simulink model "UAV_Autotune_Model_4Axis"  (R2024b)
settings: Solver=ode23t  StartTime=0.0  StopTime=55  MaxStep=0.01  RelTol=1e-3
values from neighbouring files (symbols this model uses):
  P = merge_struct_recursive(P,A.overrides)    [apply_aircraft_definition.m]    (also in uav_actuator_sfunc.m = block.DialogPrm(1).Data; uav_aero_sfunc.m = block.DialogPrm(1).Data; uav_autopilot_sfunc.m = block.DialogPrm(1).Data; uav_command_sfunc.m = block.DialogPrm(1).Data)
libraries: aerolibatmos2 x1, aerolibobsolete x1, shared6dof x1
settings Model: Creator=dell  LastModifiedBy=dell

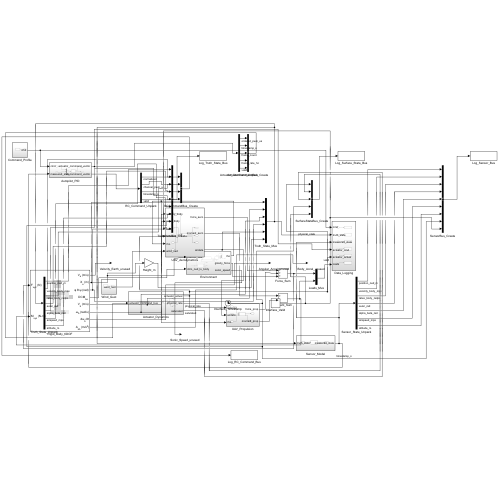
[thumbnail: Simulink's stored preview of the top-level diagram]
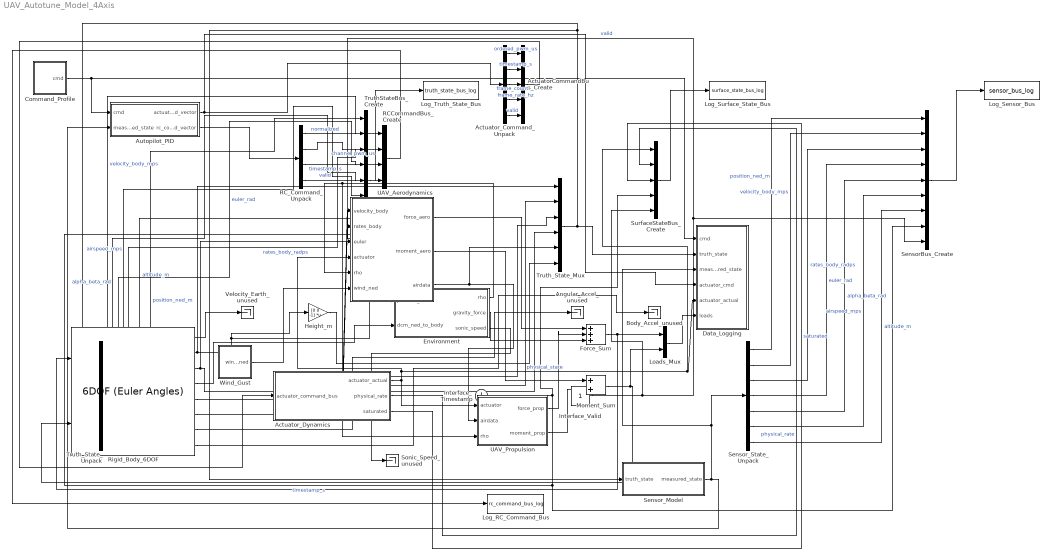
== system UAV_Autotune_Model_4Axis ==
  ActuatorCommandBus_Create : BusCreator  Inputs=5  OutDataTypeStr=Bus: ActuatorCommandBus
  Actuator_Command_Unpack : Demux  Outputs=[5 1 1 1 1]
  Actuator_Dynamics : Subsystem
  Angular_Accel_unused : Terminator
  Autopilot_PID : Subsystem
  Body_Accel_unused : Terminator
  Command_Profile : Subsystem
  Data_Logging : Subsystem
  Environment : Subsystem
  Force_Sum : Sum  Inputs=+++
  Height_m : Gain  Gain=[0 0 -1]  Multiplication=Matrix(K*u)
  Interface_Timestamp : Clock
  Interface_Valid : Constant
  Loads_Mux : Mux  Inputs=2
  Log_RC_Command_Bus : ToWorkspace  VariableName=rc_command_bus_log  SaveFormat=Timeseries  SampleTime=-1
  Log_Sensor_Bus : ToWorkspace  VariableName=sensor_bus_log  SaveFormat=Timeseries  SampleTime=-1
  Log_Surface_State_Bus : ToWorkspace  VariableName=surface_state_bus_log  SaveFormat=Timeseries  SampleTime=-1
  Log_Truth_State_Bus : ToWorkspace  VariableName=truth_state_bus_log  SaveFormat=Timeseries  SampleTime=-1
  Moment_Sum : Sum
  RCCommandBus_Create : BusCreator  Inputs=4  OutDataTypeStr=Bus: RCCommandBus
  RC_Command_Unpack : Demux  Outputs=[4 8 1 1]
  Rigid_Body_6DOF : shared6dof/6DOF (Euler Angles)  units=Metric (MKS)  mtype=Fixed  rep=Euler Angles  xme_0=P.init.position_ned  Vm_0=P.init.velocity_body  eul_0=P.init.euler  pm_0=P.init.body_rates  mass_0=P.mass  mass_e=0.5  mass_f=2.0  inertia=P.inertia  inertia_e=eye(3)  inertia_f=2*eye(3)  k_quat=1.0  vre_flag=on  abi_flag=off  aMode=aMode  xme_statename=''  Vm_statename=''  eul_statename=''  quat_statename=''  pm_statename=''  mass_statename=''
  SensorBus_Create : BusCreator  Inputs=9  OutDataTypeStr=Bus: SensorBus
  Sensor_Model : Subsystem
  Sensor_State_Unpack : Demux  Outputs=[3 3 3 3 2 1 1]
  Sonic_Speed_unused : Terminator
  SurfaceStateBus_Create : BusCreator  Inputs=5  OutDataTypeStr=Bus: SurfaceStateBus
  TruthStateBus_Create : BusCreator  Inputs=9  OutDataTypeStr=Bus: TruthStateBus
  Truth_State_Mux : Mux  Inputs=6
  Truth_State_Unpack : Demux  Outputs=[3 3 3 3 2 1 1]
  UAV_Aerodynamics : Subsystem
  UAV_Propulsion : Subsystem
  Velocity_Earth_unused : Terminator
  Wind_Gust : Subsystem
  wires:
  Loads_Mux/1 -> Data_Logging/6(loads)
  Command_Profile/1(cmd) -> Autopilot_PID/1(cmd), Data_Logging/1(cmd)
  Rigid_Body_6DOF/8 -> Body_Accel_unused/1
  Rigid_Body_6DOF/7 -> Angular_Accel_unused/1
  Rigid_Body_6DOF/1 -> Velocity_Earth_unused/1
  Rigid_Body_6DOF/3 -> Truth_State_Mux/4, UAV_Aerodynamics/3(euler)
  Rigid_Body_6DOF/6 -> Truth_State_Mux/3, UAV_Aerodynamics/2(rates_body)
  Rigid_Body_6DOF/5 -> Truth_State_Mux/2, UAV_Aerodynamics/1(velocity_body)
  Rigid_Body_6DOF/4 -> Environment/2(dcm_ned_to_body)
  Rigid_Body_6DOF/2 -> Height_m/1, Environment/1(position_ned), Truth_State_Mux/1
  Environment/1(rho) -> UAV_Aerodynamics/5(rho), UAV_Propulsion/3(rho)
  UAV_Aerodynamics/3(airdata) -> Truth_State_Mux/5, UAV_Propulsion/2(airdata)
  UAV_Aerodynamics/1(force_aero) -> Force_Sum/1
  UAV_Propulsion/1(force_prop) -> Force_Sum/2
  Environment/2(gravity_force) -> Force_Sum/3
  UAV_Aerodynamics/2(moment_aero) -> Moment_Sum/1
  UAV_Propulsion/2(moment_prop) -> Moment_Sum/2
  Height_m/1 -> Truth_State_Mux/6
  Force_Sum/1 -> Rigid_Body_6DOF/1, Loads_Mux/1
  Moment_Sum/1 -> Rigid_Body_6DOF/2, Loads_Mux/2
  Environment/3(sonic_speed) -> Sonic_Speed_unused/1
  RC_Command_Unpack/4 -> RCCommandBus_Create/4  "valid"
  RC_Command_Unpack/3 -> RCCommandBus_Create/3  "timestamp_s"
  Autopilot_PID/2(rc_command_vector) -> RC_Command_Unpack/1
  RC_Command_Unpack/1 -> RCCommandBus_Create/1  "normalized"
  RC_Command_Unpack/2 -> RCCommandBus_Create/2  "channel_pwm_us"
  SensorBus_Create/1 -> Log_Sensor_Bus/1
  Sensor_State_Unpack/7 -> SensorBus_Create/7  "altitude_m"
  Sensor_State_Unpack/6 -> SensorBus_Create/6  "airspeed_mps"
  Sensor_State_Unpack/5 -> SensorBus_Create/5  "alpha_beta_rad"
  Sensor_State_Unpack/4 -> SensorBus_Create/4  "euler_rad"
  Sensor_State_Unpack/3 -> SensorBus_Create/3  "rates_body_radps"
  Sensor_State_Unpack/2 -> SensorBus_Create/2  "velocity_body_mps"
  Sensor_State_Unpack/1 -> SensorBus_Create/1  "position_ned_m"
  TruthStateBus_Create/1 -> Log_Truth_State_Bus/1
  Truth_State_Unpack/7 -> TruthStateBus_Create/7  "altitude_m"
  Truth_State_Unpack/6 -> TruthStateBus_Create/6  "airspeed_mps"
  Truth_State_Unpack/5 -> TruthStateBus_Create/5  "alpha_beta_rad"
  Truth_State_Unpack/4 -> TruthStateBus_Create/4  "euler_rad"
  Truth_State_Unpack/3 -> TruthStateBus_Create/3  "rates_body_radps"
  Truth_State_Unpack/2 -> TruthStateBus_Create/2  "velocity_body_mps"
  Truth_State_Unpack/1 -> TruthStateBus_Create/1  "position_ned_m"
  SurfaceStateBus_Create/1 -> Log_Surface_State_Bus/1
  Interface_Valid/1 -> SensorBus_Create/9, TruthStateBus_Create/9, SurfaceStateBus_Create/5  "valid"
  Interface_Timestamp/1 -> SensorBus_Create/8, TruthStateBus_Create/8, SurfaceStateBus_Create/4  "timestamp_s"
  Actuator_Dynamics/3(saturated) -> SurfaceStateBus_Create/3  "saturated"
  Actuator_Dynamics/2(physical_rate) -> SurfaceStateBus_Create/2  "physical_rate"
  RCCommandBus_Create/1 -> Log_RC_Command_Bus/1
  ActuatorCommandBus_Create/1 -> Actuator_Dynamics/1(actuator_command_bus)
  Actuator_Command_Unpack/2 -> ActuatorCommandBus_Create/2  "timestamp_s"
  Actuator_Command_Unpack/1 -> ActuatorCommandBus_Create/1  "ordered_pwm_us"
  Actuator_Dynamics/1(actuator_actual) -> SurfaceStateBus_Create/1, Data_Logging/5(actuator_actual), UAV_Aerodynamics/4(actuator), UAV_Propulsion/1(actuator)  "physical_state"
  Autopilot_PID/1(actuator_command_vector) -> Actuator_Command_Unpack/1, Data_Logging/4(actuator_cmd)
  Actuator_Command_Unpack/3 -> ActuatorCommandBus_Create/3  "frame_count"
  Actuator_Command_Unpack/4 -> ActuatorCommandBus_Create/4  "frame_rate_hz"
  Actuator_Command_Unpack/5 -> ActuatorCommandBus_Create/5  "valid"
  Sensor_Model/1(measured_state) -> Sensor_State_Unpack/1, Data_Logging/3(measured_state), Autopilot_PID/2(measured_state)
  Truth_State_Mux/1 -> Truth_State_Unpack/1, Sensor_Model/1(truth_state), Data_Logging/2(truth_state)
  Wind_Gust/1(wind_ned) -> UAV_Aerodynamics/6(wind_ned)

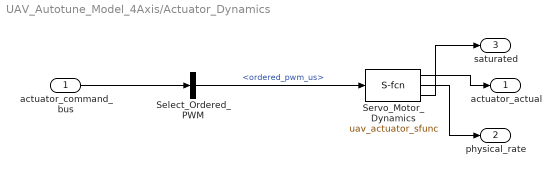
== system UAV_Autotune_Model_4Axis/Actuator_Dynamics ==
  actuator_command_bus : Inport  OutDataTypeStr=Bus: ActuatorCommandBus
  Select_Ordered_PWM : BusSelector  OutputSignals=ordered_pwm_us
  Servo_Motor_Dynamics : M-S-Function  FunctionName=uav_actuator_sfunc  Parameters=P
  actuator_actual : Outport
  physical_rate : Outport  Port=2
  saturated : Outport  Port=3
  wires:
  Select_Ordered_PWM/1 -> Servo_Motor_Dynamics/1  "<ordered_pwm_us>"
  actuator_command_bus/1 -> Select_Ordered_PWM/1
  Servo_Motor_Dynamics/1 -> actuator_actual/1
  Servo_Motor_Dynamics/3 -> saturated/1
  Servo_Motor_Dynamics/2 -> physical_rate/1

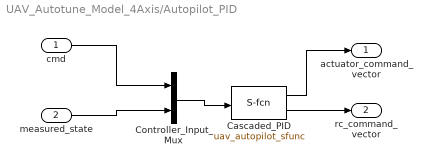
== system UAV_Autotune_Model_4Axis/Autopilot_PID ==
  cmd : Inport
  measured_state : Inport  Port=2
  Cascaded_PID : M-S-Function  FunctionName=uav_autopilot_sfunc  Parameters=P
  Controller_Input_Mux : Mux  Inputs=2
  actuator_command_vector : Outport
  rc_command_vector : Outport  Port=2
  wires:
  measured_state/1 -> Controller_Input_Mux/2
  cmd/1 -> Controller_Input_Mux/1
  Controller_Input_Mux/1 -> Cascaded_PID/1
  Cascaded_PID/2 -> rc_command_vector/1
  Cascaded_PID/1 -> actuator_command_vector/1

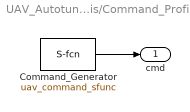
== system UAV_Autotune_Model_4Axis/Command_Profile ==
  Command_Generator : M-S-Function  FunctionName=uav_command_sfunc  Parameters=P
  cmd : Outport
  wires:
  Command_Generator/1 -> cmd/1

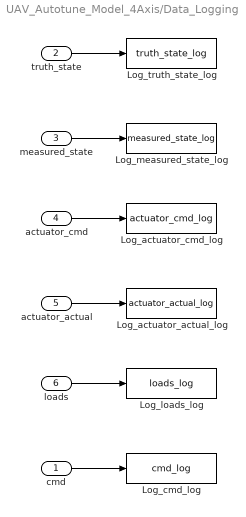
== system UAV_Autotune_Model_4Axis/Data_Logging ==
  cmd : Inport
  truth_state : Inport  Port=2
  measured_state : Inport  Port=3
  actuator_cmd : Inport  Port=4
  actuator_actual : Inport  Port=5
  loads : Inport  Port=6
  Log_actuator_actual_log : ToWorkspace  VariableName=actuator_actual_log  SaveFormat=Timeseries  SampleTime=-1
  Log_actuator_cmd_log : ToWorkspace  VariableName=actuator_cmd_log  SaveFormat=Timeseries  SampleTime=-1
  Log_cmd_log : ToWorkspace  VariableName=cmd_log  SaveFormat=Timeseries  SampleTime=-1
  Log_loads_log : ToWorkspace  VariableName=loads_log  SaveFormat=Timeseries  SampleTime=-1
  Log_measured_state_log : ToWorkspace  VariableName=measured_state_log  SaveFormat=Timeseries  SampleTime=-1
  Log_truth_state_log : ToWorkspace  VariableName=truth_state_log  SaveFormat=Timeseries  SampleTime=-1
  wires:
  loads/1 -> Log_loads_log/1
  actuator_actual/1 -> Log_actuator_actual_log/1
  actuator_cmd/1 -> Log_actuator_cmd_log/1
  measured_state/1 -> Log_measured_state_log/1
  truth_state/1 -> Log_truth_state_log/1
  cmd/1 -> Log_cmd_log/1

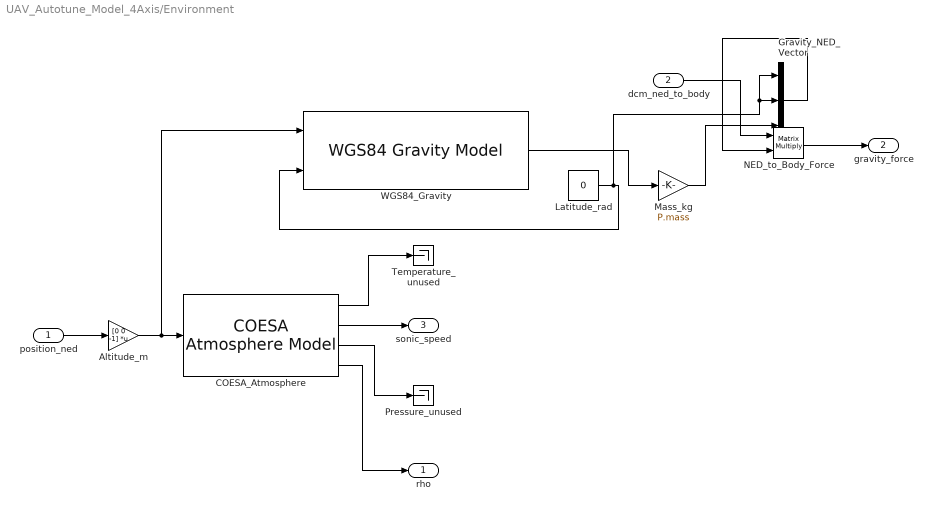
== system UAV_Autotune_Model_4Axis/Environment ==
  position_ned : Inport
  dcm_ned_to_body : Inport  Port=2
  Altitude_m : Gain  Gain=[0 0 -1]  Multiplication=Matrix(K*u)
  COESA_Atmosphere : aerolibatmos2/COESA Atmosphere Model  units=Metric (MKS)  spec=1976 COESA-extended U.S. Standard Atmosphere  model=Profile  profile_var=High temperature  profile_percent=1%  profile_alt=5 km (16404 ft)  envelope_var=High temperature  envelope_percent=1%  action=Warning
  Gravity_NED_Vector : Mux  Inputs=3
  Latitude_rad : Constant  Value=0
  Mass_kg : Gain  Gain=P.mass
  NED_to_Body_Force : Product  Inputs=**  Multiplication=Matrix(*)
  Pressure_unused : Terminator
  Temperature_unused : Terminator
  WGS84_Gravity : aerolibobsolete/WGS84 Gravity Model  model=WGS84 Taylor Series  units=Metric (MKS)  no_atmos=on  precessing=on  month=October  day=10  year=2004  no_centrifugal=on  action=Warning
  rho : Outport
  gravity_force : Outport  Port=2
  sonic_speed : Outport  Port=3
  wires:
  COESA_Atmosphere/3 -> Pressure_unused/1
  COESA_Atmosphere/1 -> Temperature_unused/1
  COESA_Atmosphere/2 -> sonic_speed/1
  NED_to_Body_Force/1 -> gravity_force/1
  COESA_Atmosphere/4 -> rho/1
  dcm_ned_to_body/1 -> NED_to_Body_Force/1
  position_ned/1 -> Altitude_m/1
  Altitude_m/1 -> WGS84_Gravity/1, COESA_Atmosphere/1
  Gravity_NED_Vector/1 -> NED_to_Body_Force/2
  Mass_kg/1 -> Gravity_NED_Vector/3
  WGS84_Gravity/1 -> Mass_kg/1
  Latitude_rad/1 -> Gravity_NED_Vector/1, Gravity_NED_Vector/2, WGS84_Gravity/2

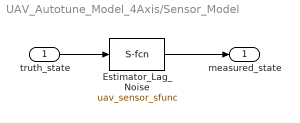
== system UAV_Autotune_Model_4Axis/Sensor_Model ==
  truth_state : Inport
  Estimator_Lag_Noise : M-S-Function  FunctionName=uav_sensor_sfunc  Parameters=P
  measured_state : Outport
  wires:
  Estimator_Lag_Noise/1 -> measured_state/1
  truth_state/1 -> Estimator_Lag_Noise/1

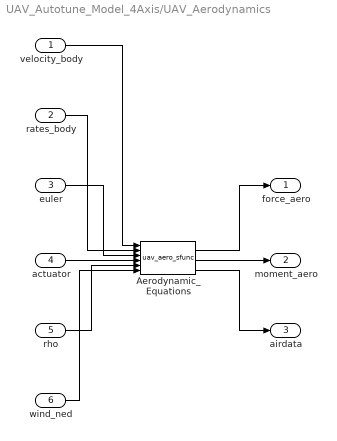
== system UAV_Autotune_Model_4Axis/UAV_Aerodynamics ==
  velocity_body : Inport
  rates_body : Inport  Port=2
  euler : Inport  Port=3
  actuator : Inport  Port=4
  rho : Inport  Port=5
  wind_ned : Inport  Port=6
  Aerodynamic_Equations : M-S-Function  FunctionName=uav_aero_sfunc  Parameters=P
  force_aero : Outport
  moment_aero : Outport  Port=2
  airdata : Outport  Port=3
  wires:
  Aerodynamic_Equations/3 -> airdata/1
  Aerodynamic_Equations/2 -> moment_aero/1
  Aerodynamic_Equations/1 -> force_aero/1
  wind_ned/1 -> Aerodynamic_Equations/6
  rho/1 -> Aerodynamic_Equations/5
  actuator/1 -> Aerodynamic_Equations/4
  euler/1 -> Aerodynamic_Equations/3
  rates_body/1 -> Aerodynamic_Equations/2
  velocity_body/1 -> Aerodynamic_Equations/1

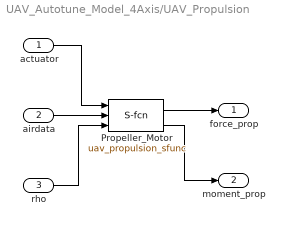
== system UAV_Autotune_Model_4Axis/UAV_Propulsion ==
  actuator : Inport
  airdata : Inport  Port=2
  rho : Inport  Port=3
  Propeller_Motor : M-S-Function  FunctionName=uav_propulsion_sfunc  Parameters=P
  force_prop : Outport
  moment_prop : Outport  Port=2
  wires:
  Propeller_Motor/2 -> moment_prop/1
  Propeller_Motor/1 -> force_prop/1
  rho/1 -> Propeller_Motor/3
  airdata/1 -> Propeller_Motor/2
  actuator/1 -> Propeller_Motor/1

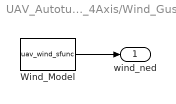
== system UAV_Autotune_Model_4Axis/Wind_Gust ==
  Wind_Model : M-S-Function  FunctionName=uav_wind_sfunc  Parameters=P
  wind_ned : Outport
  wires:
  Wind_Model/1 -> wind_ned/1
